simulink model "Hierarchical_Scheduler"  (Simulink 7.3)
settings: Solver=ode45  StartTime=0.0  StopTime=5000  RelTol=1e-3
undefined symbols (not defined in the file or in its folder): DiscIntNeverNeededParam
libraries: simulink x3
settings Model: Creator=nmd01  LastModifiedBy=nmd01

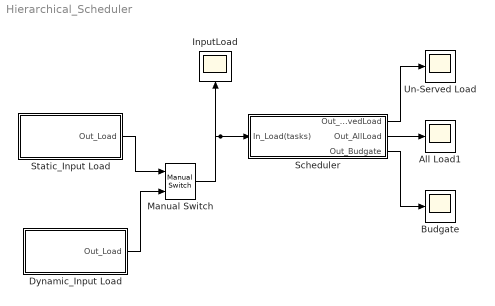
== system Hierarchical_Scheduler ==
  All Load1 : Scope
      settings: SaveName=Utilization1  DataFormat=Array
  Budgate : Scope
      settings: SaveName=Utilization2  DataFormat=Array
  Dynamic_Input Load : Subsystem
  InputLoad : Scope
      settings: SaveName=Utilization3  DataFormat=Array
  Manual Switch : simulink/Signal Routing/Manual Switch  SystemSampleTime=-1  sw=1  action=0  varsize=off
  Scheduler : Subsystem
  Static_Input Load : Subsystem
  Un-Served Load : Scope
      settings: SaveName=h  DataFormat=Array
  wires:
  Scheduler/1(Out_Un-servedLoad) -> Un-Served Load/1
  Scheduler/2(Out_AllLoad) -> All Load1/1
  Scheduler/3(Out_Budgate) -> Budgate/1
  Static_Input Load/1(Out_Load) -> Manual Switch/1
  Dynamic_Input Load/1(Out_Load) -> Manual Switch/2
  Manual Switch/1 -> Scheduler/1(In_Load(tasks)), InputLoad/1

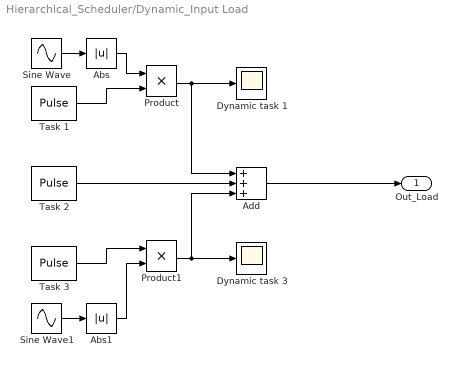
== system Hierarchical_Scheduler/Dynamic_Input Load ==
  Abs : Abs  OutDataType=fixdt(1, 16)  OutScaling=2^0
  Abs1 : Abs  OutDataType=fixdt(1, 16)  OutScaling=2^0
  Add : Sum  Inputs=+++  OutDataType=fixdt(1, 16)  OutScaling=2^-10
  Dynamic task 1 : Scope
      settings: SaveName=Utilization6  DataFormat=Array
  Dynamic task 3 : Scope
      settings: SaveName=Utilization7  DataFormat=Array
  Product : Product  OutDataType=fixdt(1, 16)  OutScaling=2^0  SampleTime=1  RndMeth=Zero
  Product1 : Product  OutDataType=fixdt(1, 16)  OutScaling=2^0  SampleTime=1  RndMeth=Zero
  Sine Wave : Sin  Amplitude=1  Bias=0  Frequency=1  Phase=0  Samples=10  SampleTime=0  Offset=0
  Sine Wave1 : Sin  Amplitude=1  Bias=0  Frequency=3  Phase=0  Samples=10  SampleTime=0  Offset=0
  Task 1 : DiscretePulseGenerator  PulseType=Time based  Amplitude=5  Period=10  PulseWidth=1  PhaseDelay=0  SampleTime=1
  Task 2 : DiscretePulseGenerator  PulseType=Time based  Amplitude=2  Period=12  PulseWidth=1  PhaseDelay=0  SampleTime=1
  Task 3 : DiscretePulseGenerator  PulseType=Time based  Amplitude=1  Period=14  PulseWidth=1  PhaseDelay=0  SampleTime=1
  Out_Load : Outport  OutDataType=fixdt(1, 16)  OutScaling=2^0
  wires:
  Add/1 -> Out_Load/1
  Task 2/1 -> Add/2
  Sine Wave/1 -> Abs/1
  Abs/1 -> Product/1
  Task 1/1 -> Product/2
  Product/1 -> Dynamic task 1/1, Add/1
  Sine Wave1/1 -> Abs1/1
  Task 3/1 -> Product1/1
  Abs1/1 -> Product1/2
  Product1/1 -> Add/3, Dynamic task 3/1

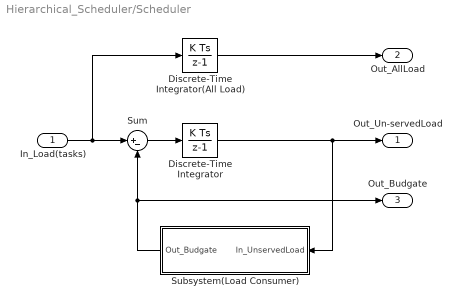
== system Hierarchical_Scheduler/Scheduler ==
  In_Load(tasks) : Inport  OutDataType=fixdt(1, 16)  OutScaling=2^0
  Discrete-Time Integrator : DiscreteIntegrator  OutDataType=fixdt(1, 16)  OutScaling=2^0  LimitOutput=on  LowerSaturationLimit=0  ICPrevOutput=DiscIntNeverNeededParam  ICPrevScaledInput=DiscIntNeverNeededParam
  Discrete-Time Integrator(All Load) : DiscreteIntegrator  OutDataType=fixdt(1, 16)  OutScaling=2^0  LimitOutput=on  LowerSaturationLimit=0  ICPrevOutput=DiscIntNeverNeededParam  ICPrevScaledInput=DiscIntNeverNeededParam
  Subsystem(Load Consumer) : Subsystem
  Sum : Sum  Inputs=|+-  OutDataType=fixdt(1, 16)  OutScaling=2^0  SampleTime=1
  Out_Un-servedLoad : Outport  OutDataType=fixdt(1, 16)  OutScaling=2^0
  Out_AllLoad : Outport  Port=2  OutDataType=fixdt(1, 16)  OutScaling=2^0
  Out_Budgate : Outport  Port=3  OutDataType=fixdt(1, 16)  OutScaling=2^0
  wires:
  In_Load(tasks)/1 -> Sum/1, Discrete-Time Integrator(All Load)/1
  Sum/1 -> Discrete-Time Integrator/1
  Discrete-Time Integrator/1 -> Out_Un-servedLoad/1, Subsystem(Load Consumer)/1(In_UnservedLoad)
  Subsystem(Load Consumer)/1(Out_Budgate) -> Sum/2, Out_Budgate/1
  Discrete-Time Integrator(All Load)/1 -> Out_AllLoad/1

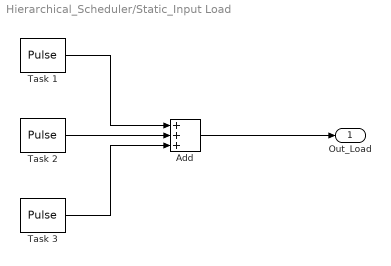
== system Hierarchical_Scheduler/Static_Input Load ==
  Add : Sum  Inputs=+++  OutDataType=fixdt(1, 16)  OutScaling=2^-10
  Task 1 : DiscretePulseGenerator  PulseType=Time based  Amplitude=3  Period=10  PulseWidth=1  PhaseDelay=0  SampleTime=1
  Task 2 : DiscretePulseGenerator  PulseType=Time based  Amplitude=2  Period=12  PulseWidth=1  PhaseDelay=0  SampleTime=1
  Task 3 : DiscretePulseGenerator  PulseType=Time based  Amplitude=1  Period=14  PulseWidth=1  PhaseDelay=0  SampleTime=1
  Out_Load : Outport  OutDataType=fixdt(1, 16)  OutScaling=2^0
  wires:
  Add/1 -> Out_Load/1
  Task 1/1 -> Add/1
  Task 2/1 -> Add/2
  Task 3/1 -> Add/3

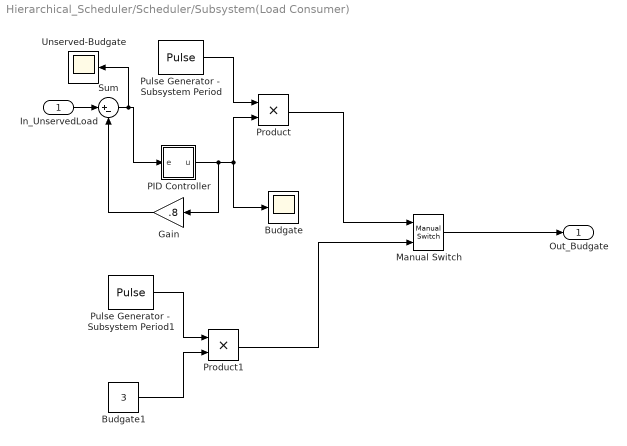
== system Hierarchical_Scheduler/Scheduler/Subsystem(Load Consumer) ==
  In_UnservedLoad : Inport  OutDataType=fixdt(1, 16)  OutScaling=2^0
  Budgate : Scope
      settings: SaveName=Utilization4  DataFormat=Array
  Budgate1 : Constant  Value=3  OutDataType=fixdt(1, 16)  OutScaling=2^0
  Gain : Gain  Gain=.8  ParameterDataType=fixdt(1, 16)  ParameterScaling=2^0  OutDataType=fixdt(1, 16)  OutScaling=2^0
  Manual Switch : simulink/Signal Routing/Manual Switch  SystemSampleTime=-1  sw=1  action=0  varsize=off
  PID Controller : Subsystem  AncestorBlock=simulink_extras/Additional Linear/PID Controller  mask(PID Controller){P=.0005, I=.0005, D=0}
      mask prompts: P "Proportional:"; I "Integral:"; D "Derivative:"
      mask help:
      | Enter expressions for proportional, integral, and derivative terms.
      | P+I/s+Ds
      mask Help: This block implements a PID controller where parameters are entered for the Proportional, Integral and Derivative terms. Unmask this block to see how it works. The derivative term is implemented using a true derivative block.
      mask Display: disp('PID')
  Product : Product  OutDataType=fixdt(1, 16)  OutScaling=2^0  SampleTime=1  RndMeth=Zero
  Product1 : Product  OutDataType=fixdt(1, 16)  OutScaling=2^0  SampleTime=1  RndMeth=Zero
  Pulse Generator -  Subsystem Period : DiscretePulseGenerator  PulseType=Time based  Amplitude=1  Period=5  PulseWidth=1  PhaseDelay=0  SampleTime=1
  Pulse Generator -  Subsystem Period1 : DiscretePulseGenerator  PulseType=Time based  Amplitude=1  Period=2  PulseWidth=1  PhaseDelay=0  SampleTime=1
  Sum : Sum  Inputs=|+-  OutDataType=fixdt(1, 16)  OutScaling=2^0  SampleTime=1
  Unserved-Budgate : Scope
      settings: SaveName=Utilization5  DataFormat=Array
  Out_Budgate : Outport  OutDataType=fixdt(1, 16)  OutScaling=2^0
  wires:
  Pulse Generator -  Subsystem Period/1 -> Product/1
  PID Controller/1(u) -> Product/2, Budgate/1, Gain/1
  In_UnservedLoad/1 -> Sum/1
  Sum/1 -> PID Controller/1(e), Unserved-Budgate/1
  Pulse Generator -  Subsystem Period1/1 -> Product1/1
  Budgate1/1 -> Product1/2
  Product/1 -> Manual Switch/1
  Product1/1 -> Manual Switch/2
  Manual Switch/1 -> Out_Budgate/1
  Gain/1 -> Sum/2

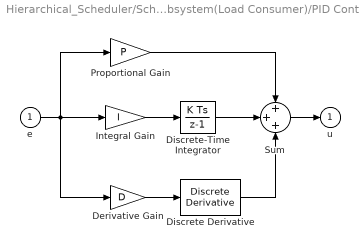
== system Hierarchical_Scheduler/Scheduler/Subsystem(Load Consumer)/PID Controller ==
  e : Inport  OutDataType=sfix(16)  OutScaling=2^0
  Derivative Gain : Gain  Gain=D  ParameterDataType=sfix(16)  ParameterScaling=2^0  OutDataType=sfix(16)  OutScaling=2^0  SampleTime=5  SaturateOnIntegerOverflow=on  OutDataTypeStr=Inherit: Same as input  ParamDataTypeStr=Inherit: Same as input
  Discrete Derivative : simulink/Discrete/Discrete Derivative  SystemSampleTime=-1  gainval=1.0  ICPrevScaledInput=0.0  OutMin=[]  OutMax=[]  OutDataType=fixdt(1, 16)  OutScaling=2^-10  DoSatur=off
  Discrete-Time Integrator : DiscreteIntegrator  InitialCondition=1.5  SampleTime=5  OutDataType=fixdt(1, 16)  OutScaling=2^0  ICPrevOutput=DiscIntNeverNeededParam  ICPrevScaledInput=DiscIntNeverNeededParam
  Integral Gain : Gain  Gain=I  ParameterDataType=sfix(16)  ParameterScaling=2^0  OutDataType=sfix(16)  OutScaling=2^0  SampleTime=5  SaturateOnIntegerOverflow=on  OutDataTypeStr=Inherit: Same as input  ParamDataTypeStr=Inherit: Same as input
  Proportional Gain : Gain  Gain=P  ParameterDataType=sfix(16)  ParameterScaling=2^0  OutDataType=sfix(16)  OutScaling=2^0  SampleTime=5  SaturateOnIntegerOverflow=on  OutDataTypeStr=Inherit: Same as input  ParamDataTypeStr=Inherit: Same as input
  Sum : Sum  Inputs=+++  OutDataType=sfix(16)  OutScaling=2^0  SaturateOnIntegerOverflow=on  InputSameDT=on  OutDataTypeStr=Inherit: Same as first input
  u : Outport  OutDataType=sfix(16)  OutScaling=2^0  InitialOutput=0
  wires:
  Integral Gain/1 -> Discrete-Time Integrator/1
  Proportional Gain/1 -> Sum/1
  Discrete-Time Integrator/1 -> Sum/2
  Discrete Derivative/1 -> Sum/3
  e/1 -> Derivative Gain/1, Proportional Gain/1, Integral Gain/1
  Sum/1 -> u/1
  Derivative Gain/1 -> Discrete Derivative/1
